simulink model "performance_DM_freq"  (R2022b)
settings: Solver=ode8  StartTime=0.0  StopTime=5.0  FixedStep=1e-6  RelTol=1e-3
settings Model: Creator=isaac  LastModifiedBy=isaac

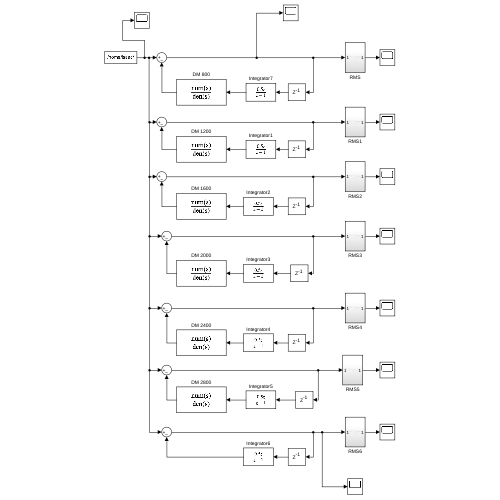
[thumbnail: Simulink's stored preview of the top-level diagram]
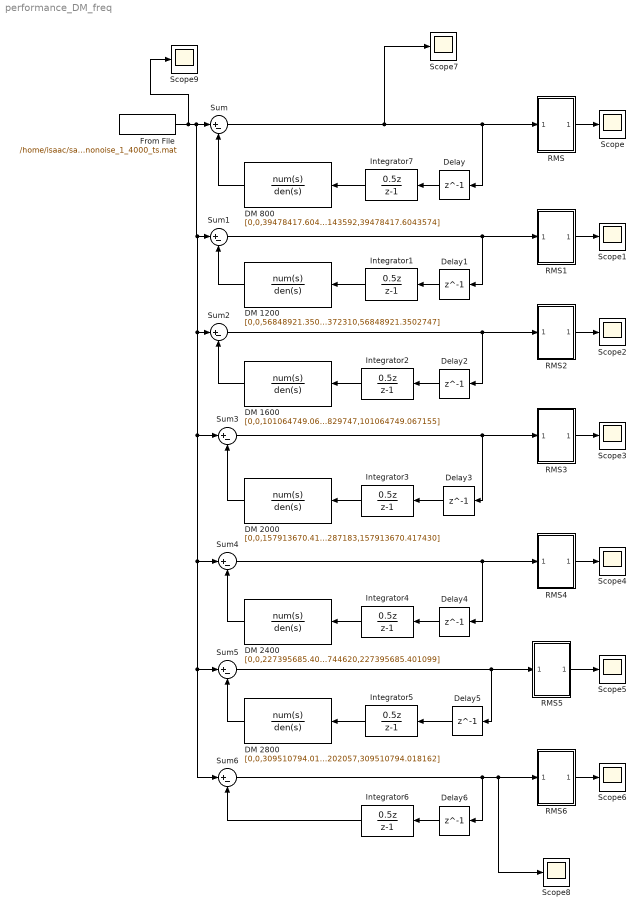
== system performance_DM_freq ==
  DM 1200 : TransferFcn  Tag=DM  Numerator=[0,0,56848921.3502747]  Denominator=[1,1507.96447372310,56848921.3502747]
  DM 1600 : TransferFcn  Tag=DM  Numerator=[0,0,101064749.067155]  Denominator=[1,2010.61929829747,101064749.067155]
  DM 2000 : TransferFcn  Tag=DM  Numerator=[0,0,157913670.417430]  Denominator=[1,2513.27412287183,157913670.417430]
  DM 2400 : TransferFcn  Tag=DM  Numerator=[0,0,227395685.401099]  Denominator=[1,3015.92894744620,227395685.401099]
  DM 2800 : TransferFcn  Tag=DM  Numerator=[0,0,309510794.018162]  Denominator=[1,3518.58377202057,309510794.018162]
  DM 800 : TransferFcn  Tag=DM  Numerator=[0,0,39478417.6043574]  Denominator=[1,1256.63706143592,39478417.6043574]
  Delay{,1..6} (7 alike) : Delay  DelayLength=1  SampleTime=0.001
  From File : FromFile  FileName=/home/isaac/saxo-plus/Data-Driven-Control-for-AO/DM_dyn/simulink/single_mode_dist_nonoise_1_4000_ts.mat  SampleTime=0.00025
  Integrator{1..7} (7 alike) : DiscreteTransferFcn  Numerator=[0.5 0]  Denominator=[1 -1]  SampleTime=0.001
  RMS : Subsystem
  RMS1 : Subsystem
  RMS2 : Subsystem
  RMS3 : Subsystem
  RMS4 : Subsystem
  RMS5 : Subsystem
  RMS6 : Subsystem
  Scope{,1..9} (10 alike) : Scope
  Sum{,1..6} (7 alike) : Sum  Inputs=|+-
  wires:
  Delay/1 -> Integrator7/1
  From File/1 -> Scope9/1, Sum6/1, Sum5/1, Sum4/1, Sum3/1, Sum2/1, Sum1/1, Sum/1
  DM 800/1 -> Sum/2
  DM 1200/1 -> Sum1/2
  DM 1600/1 -> Sum2/2
  DM 2000/1 -> Sum3/2
  DM 2400/1 -> Sum4/2
  DM 2800/1 -> Sum5/2
  Integrator7/1 -> DM 800/1
  Integrator1/1 -> DM 1200/1
  Integrator2/1 -> DM 1600/1
  Integrator3/1 -> DM 2000/1
  Integrator4/1 -> DM 2400/1
  Integrator5/1 -> DM 2800/1
  Delay2/1 -> Integrator2/1
  Delay1/1 -> Integrator1/1
  Delay3/1 -> Integrator3/1
  Delay4/1 -> Integrator4/1
  Delay5/1 -> Integrator5/1
  Sum/1 -> Scope7/1, Delay/1, RMS/1(In1)
  Sum1/1 -> Delay1/1, RMS1/1(In1)
  Sum2/1 -> Delay2/1, RMS2/1(In1)
  Sum3/1 -> Delay3/1, RMS3/1(In1)
  Sum4/1 -> Delay4/1, RMS4/1(In1)
  Sum5/1 -> Delay5/1, RMS5/1(In1)
  RMS/1(Out1) -> Scope/1
  RMS1/1(Out1) -> Scope1/1
  RMS2/1(Out1) -> Scope2/1
  RMS3/1(Out1) -> Scope3/1
  RMS4/1(Out1) -> Scope4/1
  RMS5/1(Out1) -> Scope5/1
  Integrator6/1 -> Sum6/2
  Delay6/1 -> Integrator6/1
  RMS6/1(Out1) -> Scope6/1
  Sum6/1 -> Delay6/1, RMS6/1(In1), Scope8/1

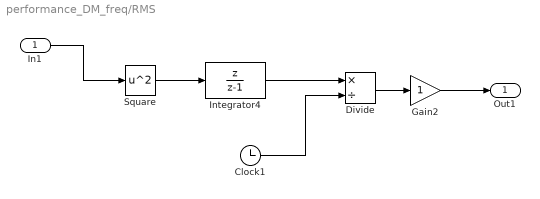
== system performance_DM_freq/RMS ==
  In1 : Inport
  Clock1 : Clock
  Divide : Product  Inputs=*/
  Gain2 : Gain
  Integrator4 : DiscreteTransferFcn  Numerator=[1 0]  Denominator=[1 -1]  SampleTime=0.00025
  Square : Math  Operator=square
  Out1 : Outport
  wires:
  Divide/1 -> Gain2/1
  Integrator4/1 -> Divide/1
  Square/1 -> Integrator4/1
  Clock1/1 -> Divide/2
  In1/1 -> Square/1
  Gain2/1 -> Out1/1

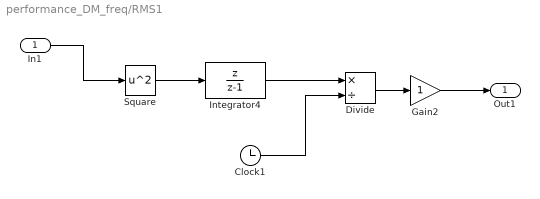
== system performance_DM_freq/RMS1 ==
  In1 : Inport
  Clock1 : Clock
  Divide : Product  Inputs=*/
  Gain2 : Gain
  Integrator4 : DiscreteTransferFcn  Numerator=[1 0]  Denominator=[1 -1]  SampleTime=0.00025
  Square : Math  Operator=square
  Out1 : Outport
  wires:
  Divide/1 -> Gain2/1
  Integrator4/1 -> Divide/1
  Square/1 -> Integrator4/1
  Clock1/1 -> Divide/2
  In1/1 -> Square/1
  Gain2/1 -> Out1/1

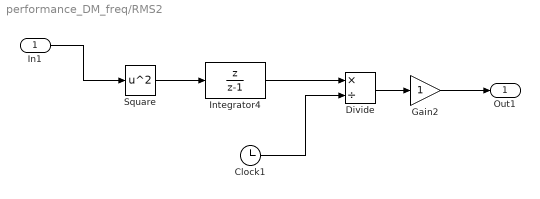
== system performance_DM_freq/RMS2 ==
  In1 : Inport
  Clock1 : Clock
  Divide : Product  Inputs=*/
  Gain2 : Gain
  Integrator4 : DiscreteTransferFcn  Numerator=[1 0]  Denominator=[1 -1]  SampleTime=0.00025
  Square : Math  Operator=square
  Out1 : Outport
  wires:
  Divide/1 -> Gain2/1
  Integrator4/1 -> Divide/1
  Square/1 -> Integrator4/1
  Clock1/1 -> Divide/2
  In1/1 -> Square/1
  Gain2/1 -> Out1/1

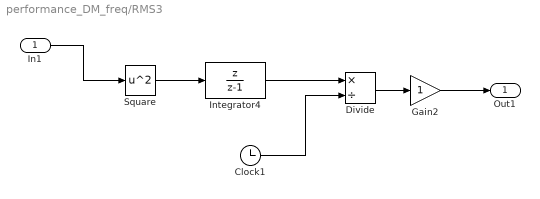
== system performance_DM_freq/RMS3 ==
  In1 : Inport
  Clock1 : Clock
  Divide : Product  Inputs=*/
  Gain2 : Gain
  Integrator4 : DiscreteTransferFcn  Numerator=[1 0]  Denominator=[1 -1]  SampleTime=0.00025
  Square : Math  Operator=square
  Out1 : Outport
  wires:
  Divide/1 -> Gain2/1
  Integrator4/1 -> Divide/1
  Square/1 -> Integrator4/1
  Clock1/1 -> Divide/2
  In1/1 -> Square/1
  Gain2/1 -> Out1/1

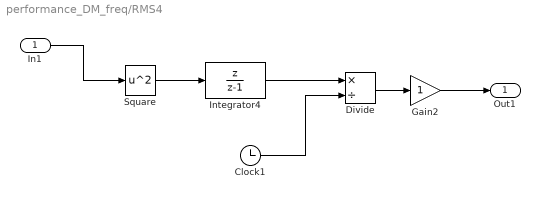
== system performance_DM_freq/RMS4 ==
  In1 : Inport
  Clock1 : Clock
  Divide : Product  Inputs=*/
  Gain2 : Gain
  Integrator4 : DiscreteTransferFcn  Numerator=[1 0]  Denominator=[1 -1]  SampleTime=0.00025
  Square : Math  Operator=square
  Out1 : Outport
  wires:
  Divide/1 -> Gain2/1
  Integrator4/1 -> Divide/1
  Square/1 -> Integrator4/1
  Clock1/1 -> Divide/2
  In1/1 -> Square/1
  Gain2/1 -> Out1/1

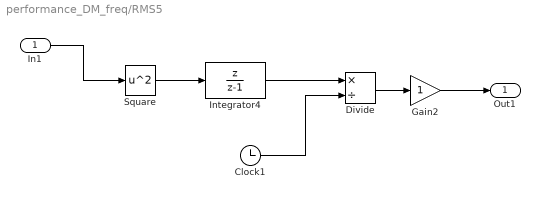
== system performance_DM_freq/RMS5 ==
  In1 : Inport
  Clock1 : Clock
  Divide : Product  Inputs=*/
  Gain2 : Gain
  Integrator4 : DiscreteTransferFcn  Numerator=[1 0]  Denominator=[1 -1]  SampleTime=0.00025
  Square : Math  Operator=square
  Out1 : Outport
  wires:
  Divide/1 -> Gain2/1
  Integrator4/1 -> Divide/1
  Square/1 -> Integrator4/1
  Clock1/1 -> Divide/2
  In1/1 -> Square/1
  Gain2/1 -> Out1/1

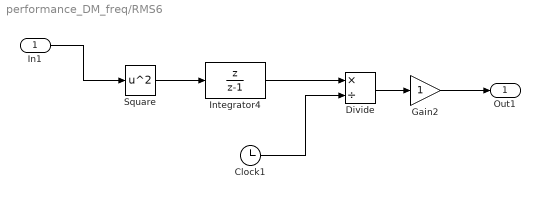
== system performance_DM_freq/RMS6 ==
  In1 : Inport
  Clock1 : Clock
  Divide : Product  Inputs=*/
  Gain2 : Gain
  Integrator4 : DiscreteTransferFcn  Numerator=[1 0]  Denominator=[1 -1]  SampleTime=0.00025
  Square : Math  Operator=square
  Out1 : Outport
  wires:
  Divide/1 -> Gain2/1
  Integrator4/1 -> Divide/1
  Square/1 -> Integrator4/1
  Clock1/1 -> Divide/2
  In1/1 -> Square/1
  Gain2/1 -> Out1/1
